simulink model "chap13_2sim"  (Simulink 8.3)
settings: Solver=ode45  StartTime=0.0  StopTime=30  FixedStep=0.001  RelTol=1e-3
settings Model: Creator=ljk  LastModifiedBy=Administrator  ExtModeTrigMode=oneshot  ExtModeArmWhenConnect=off
settings SolverCC: ZeroCrossControl=EnableAll
settings DataIOCC: LimitDataPoints=off  SignalLoggingName=sigsOut
settings OptimizationCC: BooleanDataType=off  ExpressionDepthLimit=2147483647
settings DebuggingCC: SaveWithParameterizedLinksMsg=none  SignalResolutionControl=TryResolveAllWithWarning  SolverPrmCheckMsg=none  MultiTaskDSMMsg=warning  MultiTaskCondExecSysMsg=none  FcnCallInpInsideContextMsg=UseLocalSettings
settings HardwareCC: TargetUnknown=on
settings RTWCC: IncludeERTFirstTime=on

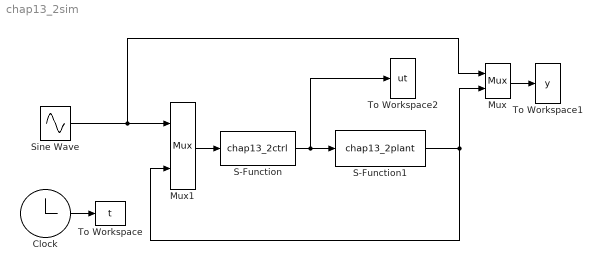
== system chap13_2sim ==
  Clock : Clock
  Mux : Mux  Inputs=2
  Mux1 : Mux  Inputs=2
  S-Function : S-Function  FunctionName=chap13_2ctrl  EnableBusSupport=off
  S-Function1 : S-Function  FunctionName=chap13_2plant  EnableBusSupport=off
  Sine Wave : Sin  SampleTime=0
  To Workspace : ToWorkspace  VariableName=t  SampleTime=-1
  To Workspace1 : ToWorkspace  VariableName=y  SampleTime=-1
  To Workspace2 : ToWorkspace  VariableName=ut  SampleTime=-1
  wires:
  Mux1/1 -> S-Function/1
  S-Function/1 -> S-Function1/1, To Workspace2/1
  Sine Wave/1 -> Mux/1, Mux1/1
  Mux/1 -> To Workspace1/1
  S-Function1/1 -> Mux1/2, Mux/2
  Clock/1 -> To Workspace/1
